simulink model "project_2_2"  (R2020a)
settings: Solver=VariableStepAuto  StartTime=0.0  StopTime=10.0  RelTol=1e-3
values from neighbouring files (symbols this model uses):
  A = 3    [project2_2.m]
  F = 2    [project2_2.m]    (also in project_3m.m = 1)
  Ti = 0.5    [project2_2.m]
settings Model: Creator=Matt  LastModifiedBy=Matt
settings DataIOCC: ReturnWorkspaceOutputs=off

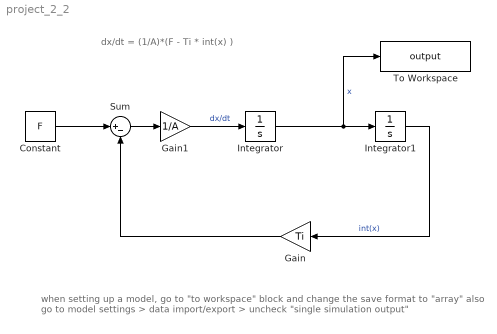
== system project_2_2 ==
  note: when setting up a model, go to "to workspace" block and change the save format to "array"
      | also go to model settings > data import/export > uncheck "single simulation output"
  note: dx/dt = (1/A)*(F - Ti * int(x) )
  Constant : Constant  Value=F
  Gain : Gain  Gain=Ti
  Gain1 : Gain  Gain=1/A
  Integrator : Integrator
  Integrator1 : Integrator
  Sum : Sum  Inputs=|+-
  To Workspace : ToWorkspace  VariableName=output  SampleTime=-1
  wires:
  Integrator/1 -> To Workspace/1, Integrator1/1  "x"
  Sum/1 -> Gain1/1
  Integrator1/1 -> Gain/1  "int(x)"
  Constant/1 -> Sum/1
  Gain/1 -> Sum/2
  Gain1/1 -> Integrator/1  "dx/dt"
